simulink model "ContinuoDiscreto_ejemplo"  (Simulink 7.1)
settings: Solver=ode45  StartTime=0.0  StopTime=10.0  RelTol=1e-3
settings Model: Creator=Usuario  LastModifiedBy=Usuario

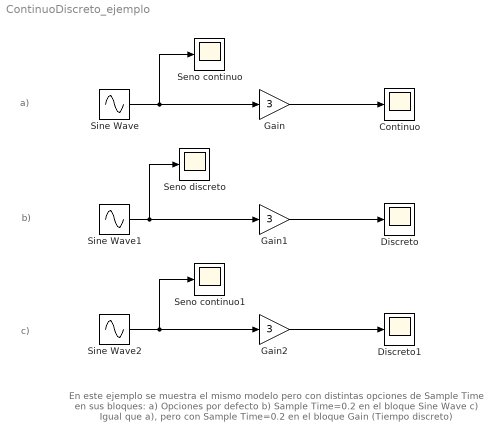
== system ContinuoDiscreto_ejemplo ==
  note: En este ejemplo se muestra el mismo modelo pero con distintas opciones de Sample Time en sus bloques:
      | a) Opciones por defecto
      | b) Sample Time=0.2 en el bloque Sine Wave
      | c) Igual que a), pero con Sample Time=0.2 en el bloque Gain (Tiempo discreto)
  note: a)
  note: b)
  note: c)
  Continuo : Scope
  Discreto : Scope
  Discreto1 : Scope
      settings: SaveName=ScopeData4
  Gain : Gain  Gain=3  ParameterDataType=sfix(16)  ParameterScaling=2^0  OutDataType=sfix(16)  OutScaling=2^0
  Gain1 : Gain  Gain=3  ParameterDataType=sfix(16)  ParameterScaling=2^0  OutDataType=sfix(16)  OutScaling=2^0
  Gain2 : Gain  Gain=3  ParameterDataType=sfix(16)  ParameterScaling=2^0  OutDataType=sfix(16)  OutScaling=2^0  SampleTime=0.2
  Seno continuo : Scope
      settings: SaveName=ScopeData2
  Seno continuo1 : Scope
      settings: SaveName=ScopeData5
  Seno discreto : Scope
      settings: SaveName=ScopeData3
  Sine Wave : Sin  SampleTime=0
  Sine Wave1 : Sin  SampleTime=0.2
  Sine Wave2 : Sin  SampleTime=0
  wires:
  Sine Wave/1 -> Seno continuo/1, Gain/1
  Gain/1 -> Continuo/1
  Sine Wave1/1 -> Seno discreto/1, Gain1/1
  Gain1/1 -> Discreto/1
  Sine Wave2/1 -> Seno continuo1/1, Gain2/1
  Gain2/1 -> Discreto1/1
